simulink model "Project_Task1_4328802_SinghShrestha"  (Simulink 8.0)
settings: Solver=ode45  StartTime=0.0  StopTime=180*Ts  RelTol=1e-3
PreLoadFcn:
  | Ts=20e-9; % Sample period
  | W=9;        % Bit-width
  | 
  | n_constant = 109;
  | gap = 300;
  | 
  | % Input sequence for n signal
  | n_value = [0 n_constant zeros(1,gap)]';   %value
  | n_time = [0:length(n_value)-1]'*Ts;          % time
  | n = [n_time n_value];                                % signal
  | 
  | % Input sequence for start signal
  | start_value = [0 1 zeros(1,gap)]';                 % value
  | start_time = [0:length(start_value)-1]'*Ts;  % time
  | start = [start_time start_value];                  % signal
undefined symbols (not defined in the file): xlipgetpartsetting
libraries: xbsIndex_r4 x37
settings Model: Creator=alpha  LastModifiedBy=SaGuN MS
settings DataIOCC: SignalLoggingSaveFormat=ModelDataLogs
settings OptimizationCC: InitFltsAndDblsToZero=on
settings DebuggingCC: SaveWithParameterizedLinksMsg=none  SignalResolutionControl=TryResolveAllWithWarning  MultiTaskDSMMsg=warning  MultiTaskCondExecSysMsg=none  FcnCallInpInsideContextMsg=EnableAllAsWarning  StrictBusMsg=Warning
settings RTWCC: IncludeERTFirstTime=on
settings GRTTargetCC: TargetFcnLib=ansi_tfl_tmw.mat  CombineOutputUpdateFcns=off  GRTInterface=on

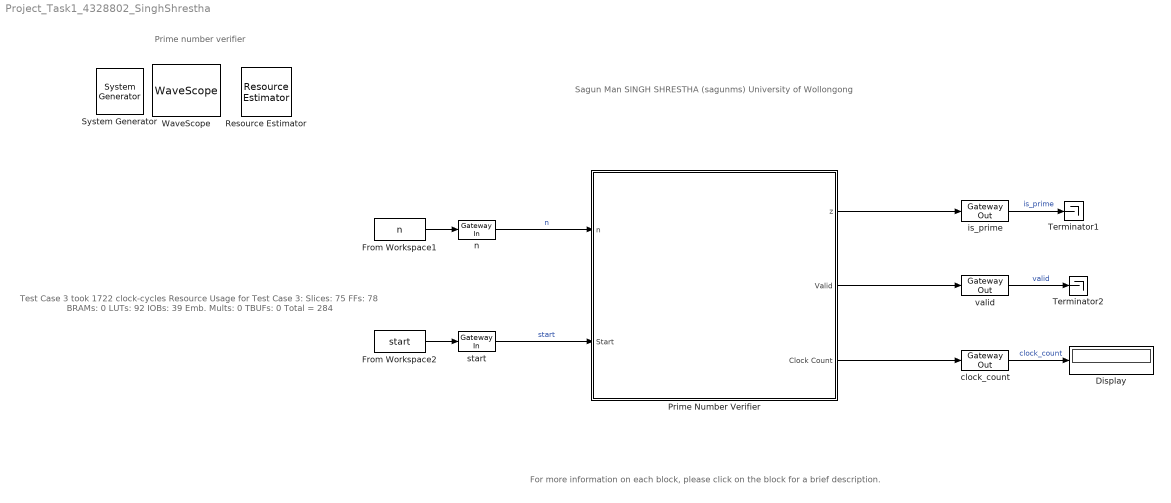
== system Project_Task1_4328802_SinghShrestha ==
  note: Prime number verifier
  note: Sagun Man SINGH SHRESTHA
      | (sagunms)
      | University of Wollongong
  note: Test Case 3 took 1722 clock-cycles
      |
      | Resource Usage for Test Case 3:
      | Slices: 75
      | FFs: 78
      | BRAMs: 0
      | LUTs: 92
      | IOBs: 39
      | Emb. Mults: 0
      | TBUFs: 0
      | Total = 284
  note: For more information on each block, please click on the block for a brief description.
  " System Generator" : xbsIndex_r4/ System Generator  Tag=genX  xilinxfamily=spartan3e  part=xc3s500e  speed=-4  package=fg320  synthesis_tool=XST  clock_wrapper=Clock Enables  directory=./ise  proj_type=Project Navigator  Synth_file=XST Defaults  Impl_file=ISE Defaults  testbench=off  simulink_period=Ts  sysclk_period=20  dcm_input_clock_period=100  incr_netlist=off  trim_vbits=Everywhere in SubSystem  dbl_ovrd=According to Block Masks  core_generation=According to Block Masks  run_coregen=off  deprecated_control=off  eval_field=0  block_type=sysgen
      settings: block_version=8.2.02
  Display : Display
  From Workspace1 : FromWorkspace  VariableName=n  SampleTime=Ts  Interpolate=off  OutputAfterFinalValue=Holding final value
  From Workspace2 : FromWorkspace  VariableName=start  SampleTime=Ts  Interpolate=off  OutputAfterFinalValue=Holding final value
  Prime Number Verifier : Subsystem
  Resource Estimator : xbsIndex_r4/Resource Estimator  Tag=resEstTag  Slices=75  FFs=78  BRAMs=0  LUTs=92  IOBs=39  EBMs=0  TBUFs=0  xl_use_estimator_area=off  est_options=Estimate  xl_estimator_area="[ 75  78   0  92  39   0   0 ]"  block_type=resource_estimator
      settings: AttributesFormatString=Resource\nEstimator  block_version=11.4
  Terminator1 : Terminator
  Terminator2 : Terminator
  WaveScope : xbsIndex_r4/WaveScope  block_type=wavescope
      settings: block_version=8.2.02
  clock_count : xbsIndex_r4/Gateway Out  inherit_from_input=off  hdl_port=on  timing_constraint=None  locs_specified=off  LOCs={'F9'}  UseAsDAC=off  DACChannel='1'  block_type=gatewayout
      settings: infoedit="Gateway out block.  Converts Xilinx fixed point inputs into ouputs of type Simulink integer, double, or fixed point.<P><P>Hardware notes:  In hardware these blocks become top level output ports or are discarded, depending on how they are configured."  xl_area=[0 0 0 0 24 0 0]  block_version=8.2.02
  is_prime : xbsIndex_r4/Gateway Out  inherit_from_input=off  hdl_port=on  timing_constraint=None  locs_specified=off  LOCs={'F9'}  UseAsDAC=off  DACChannel='1'  block_type=gatewayout
      settings: infoedit="Gateway out block.  Converts Xilinx fixed point inputs into ouputs of type Simulink integer, double, or fixed point.<P><P>Hardware notes:  In hardware these blocks become top level output ports or are discarded, depending on how they are configured."  xl_area=[0 0 0 0 1 0 0]  block_version=8.2.02
  n : xbsIndex_r4/Gateway In  gui_display_data_type=Fixed-point  arith_type=Unsigned  n_bits=W  bin_pt=0  preci_type=Single  exp_width=8  frac_width=24  quantization="Round  (unbiased: +/- Inf)"  overflow=Wrap  period=Ts  dbl_ovrd=off  timing_constraint=None  locs_specified=off  LOCs={'V16'}  UseAsADC=off  ADCChannel='1'  inherit_from_input=off  hdl_port=on  block_type=gatewayin
      settings: infoedit="Gateway in block.  Converts inputs of type Simulink integer, double and fixed point to  Xilinx fixed point type.<br><br>Hardware notes:  In hardware these blocks become top level input ports."  xl_area=[0 0 0 0 12 0 0]  block_version=8.2.02
  start : xbsIndex_r4/Gateway In  gui_display_data_type=Fixed-point  arith_type=Boolean  n_bits=W  bin_pt=0  preci_type=Single  exp_width=8  frac_width=24  quantization="Round  (unbiased: +/- Inf)"  overflow=Wrap  period=Ts  dbl_ovrd=off  timing_constraint=None  locs_specified=off  LOCs={'V16'}  UseAsADC=off  ADCChannel='1'  inherit_from_input=off  hdl_port=on  block_type=gatewayin
      settings: infoedit="Gateway in block.  Converts inputs of type Simulink integer, double and fixed point to  Xilinx fixed point type.<P><P>Hardware notes:  In hardware these blocks become top level input ports."  xl_area=[0 0 0 0 1 0 0]  block_version=8.2.02
  valid : xbsIndex_r4/Gateway Out  inherit_from_input=off  hdl_port=on  timing_constraint=None  locs_specified=off  LOCs={'F9'}  UseAsDAC=off  DACChannel='1'  block_type=gatewayout
      settings: infoedit="Gateway out block.  Converts Xilinx fixed point inputs into ouputs of type Simulink integer, double, or fixed point.<P><P>Hardware notes:  In hardware these blocks become top level output ports or are discarded, depending on how they are configured."  xl_area=[0 0 0 0 1 0 0]  block_version=8.2.02
  wires:
  From Workspace1/1 -> n/1
  From Workspace2/1 -> start/1
  is_prime/1 -> Terminator1/1  "is_prime"
  valid/1 -> Terminator2/1  "valid"
  clock_count/1 -> Display/1  "clock_count"
  n/1 -> Prime Number Verifier/1(n)  "n"
  start/1 -> Prime Number Verifier/2(Start)  "start"
  Prime Number Verifier/1(z) -> is_prime/1
  Prime Number Verifier/2(Valid) -> valid/1
  Prime Number Verifier/3(Clock Count) -> clock_count/1

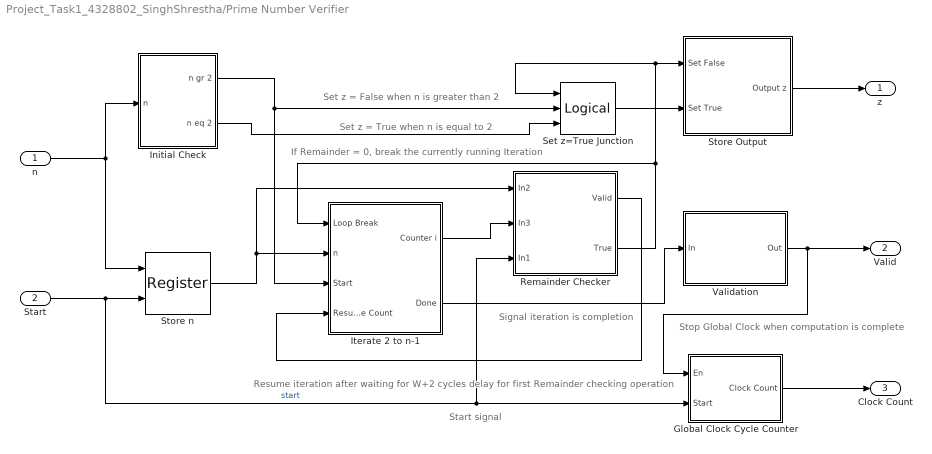
== system Project_Task1_4328802_SinghShrestha/Prime Number Verifier ==
  note: Start signal
  note: Set z = False when n is greater than 2
  note: Set z = True when n is equal to 2
  note: Signal iteration is completion
  note: If Remainder = 0, break the currently running Iteration
  note: Resume iteration after waiting for W+2 cycles delay for first Remainder checking operation
  note: Stop Global Clock when computation is complete
  n : Inport
  Start : Inport  Port=2
  Global Clock Cycle Counter : Subsystem
  Initial Check : Subsystem
  Iterate 2 to n-1 : Subsystem
  Remainder Checker : Subsystem
  Set z=True Junction : xbsIndex_r4/Logical  logical_function=OR  inputs=3  en=off  latency=0  precision=Full  arith_type=Unsigned  n_bits=16  bin_pt=0  align_bp=on  dbl_ovrd=off  block_type=logical
      settings: xl_area=[1 0 0 1 0 0 0]
  Store Output : Subsystem
  Store n : xbsIndex_r4/Register  init=0  rst=off  en=on  dbl_ovrd=off  block_type=register
      settings: xl_area=[6 12 0 0 0 0 0]
  Validation : Subsystem
  z : Outport
  Valid : Outport  Port=2
  Clock Count : Outport  Port=3
  wires:
  Start/1 -> Global Clock Cycle Counter/2(Start), Remainder Checker/3(In1), Store n/2  "start"
  n/1 -> Store n/1, Initial Check/1(n)
  Store n/1 -> Remainder Checker/1(In2), Iterate 2 to n-1/2(n)
  Validation/1(Out) -> Global Clock Cycle Counter/1(En), Valid/1
  Global Clock Cycle Counter/1(Clock Count) -> Clock Count/1
  Initial Check/1(n gr 2) -> Set z=True Junction/2, Iterate 2 to n-1/3(Start)
  Store Output/1(Output z) -> z/1
  Initial Check/2(n eq 2) -> Set z=True Junction/3
  Set z=True Junction/1 -> Store Output/2(Set True)
  Iterate 2 to n-1/2(Done) -> Validation/1(In)
  Remainder Checker/2(True) -> Store Output/1(Set False), Set z=True Junction/1, Iterate 2 to n-1/1(Loop Break)
  Iterate 2 to n-1/1(Counter i) -> Remainder Checker/2(In3)
  Remainder Checker/1(Valid) -> Iterate 2 to n-1/4(Resume Count)

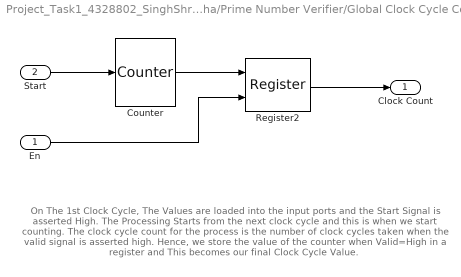
== system Project_Task1_4328802_SinghShrestha/Prime Number Verifier/Global Clock Cycle Counter ==
  note: On The 1st Clock Cycle, The Values are loaded into the input ports and the Start Signal is asserted High.
      |
      | The Processing Starts from the next clock cycle and this is when we start counting.
      | The clock cycle count for the process is the number of clock cycles taken when the valid signal is asserted high.
      |
      | Hence, we store the value of the counter when Valid=High in a register and This becomes our final Clock Cycle Value.
  En : Inport
  Start : Inport  Port=2
  Counter : xbsIndex_r4/Counter  cnt_type=Free Running  cnt_to=Inf  operation=Up  start_count=1  cnt_by_val=1  arith_type=Unsigned  n_bits=2*W  bin_pt=0  load_pin=off  rst=on  en=off  explicit_period=off  period=1  dbl_ovrd=off  use_behavioral_HDL=off  implementation=Fabric  use_rpm=off  block_type=counter
      settings: xl_area=[13 24 0 24 0 0 0]  block_version=8.2.02
  Register2 : xbsIndex_r4/Register  init=0  rst=off  en=on  dbl_ovrd=off  block_type=register
      settings: xl_area=[12 24 0 0 0 0 0]  block_version=11.4
  Clock Count : Outport
  wires:
  Counter/1 -> Register2/1
  Register2/1 -> Clock Count/1
  Start/1 -> Counter/1
  En/1 -> Register2/2

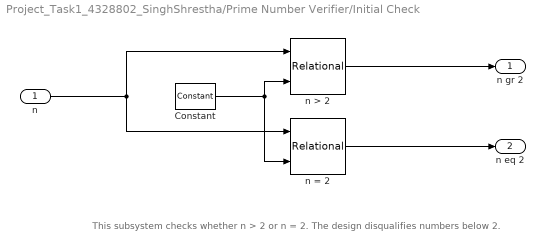
== system Project_Task1_4328802_SinghShrestha/Prime Number Verifier/Initial Check ==
  note: This subsystem checks whether n > 2 or n = 2. The design disqualifies numbers below 2.
  n : Inport
  Constant : xbsIndex_r4/Constant  const=2  gui_display_data_type=Fixed-point  arith_type=Unsigned  n_bits=2  bin_pt=0  preci_type=Single  exp_width=8  frac_width=24  explicit_period=off  period=1  equ=P=C  opselect=C  inp2=PCIN>>17  opr=+  inp1=P  carry=CIN  dbl_ovrd=off  block_type=constant
  n = 2 : xbsIndex_r4/Relational  mode=a=b  en=off  latency=0  dbl_ovrd=off  block_type=relational
      settings: xl_area=[3 0 0 6 0 0 0]
  n > 2 : xbsIndex_r4/Relational  mode=a>b  en=off  latency=0  dbl_ovrd=off  block_type=relational
      settings: xl_area=[6 0 0 12 0 0 0]
  n gr 2 : Outport
  n eq 2 : Outport  Port=2
  wires:
  n > 2/1 -> n gr 2/1
  Constant/1 -> n > 2/2, n = 2/2
  n = 2/1 -> n eq 2/1
  n/1 -> n > 2/1, n = 2/1

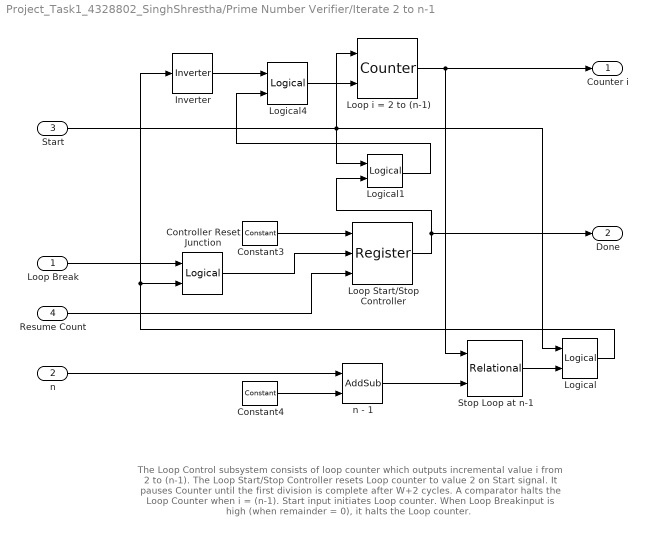
== system Project_Task1_4328802_SinghShrestha/Prime Number Verifier/Iterate 2 to n-1 ==
  note: The Loop Control subsystem consists of loop counter which outputs incremental value i from 2 to (n-1).
      | The Loop Start/Stop Controller resets Loop counter to value 2 on Start signal. It pauses Counter until the first division is complete after W+2 cycles.
      | A comparator halts the Loop Counter when i = (n-1).
      |
      | Start input initiates Loop counter. When Loop Breakinput is high (when remainder = 0), it halts the Loop counter.
  Loop Break : Inport
  n : Inport  Port=2
  Start : Inport  Port=3
  Resume Count : Inport  Port=4
  Constant3 : xbsIndex_r4/Constant  const=1  gui_display_data_type=Boolean  arith_type=Boolean  n_bits=16  bin_pt=14  preci_type=Single  exp_width=8  frac_width=24  explicit_period=off  period=1  equ=P=C  opselect=C  inp2=PCIN>>17  opr=+  inp1=P  carry=CIN  dbl_ovrd=off  block_type=constant
  Constant4 : xbsIndex_r4/Constant  const=1  gui_display_data_type=Fixed-point  arith_type=Unsigned  n_bits=W  bin_pt=0  preci_type=Single  exp_width=8  frac_width=24  explicit_period=off  period=1  equ=P=C  opselect=C  inp2=PCIN>>17  opr=+  inp1=P  carry=CIN  dbl_ovrd=off  block_type=constant
  Controller Reset Junction : xbsIndex_r4/Logical  logical_function=OR  inputs=2  en=off  latency=0  precision=Full  arith_type=Unsigned  n_bits=16  bin_pt=0  align_bp=on  dbl_ovrd=off  block_type=logical
      settings: xl_area=[1 0 0 1 0 0 0]
  Inverter : xbsIndex_r4/Inverter  en=off  latency=0  dbl_ovrd=off  block_type=inv
      settings: xl_area=[0 0 0 0 0 0 0]
  Logical : xbsIndex_r4/Logical  logical_function=NOR  inputs=2  en=off  latency=0  precision=Full  arith_type=Unsigned  n_bits=16  bin_pt=0  align_bp=on  dbl_ovrd=off  block_type=logical
      settings: xl_area=[1 0 0 1 0 0 0]
  Logical1 : xbsIndex_r4/Logical  logical_function=OR  inputs=2  en=off  latency=0  precision=Full  arith_type=Unsigned  n_bits=16  bin_pt=0  align_bp=on  dbl_ovrd=off  block_type=logical
      settings: xl_area=[1 0 0 1 0 0 0]
  Logical4 : xbsIndex_r4/Logical  logical_function=AND  inputs=2  en=off  latency=0  precision=Full  arith_type=Unsigned  n_bits=16  bin_pt=0  align_bp=on  dbl_ovrd=off  block_type=logical
      settings: xl_area=[1 0 0 1 0 0 0]
  Loop Start/Stop Controller : xbsIndex_r4/Register  init=0  rst=on  en=on  dbl_ovrd=off  block_type=register
      settings: xl_area=[1 1 0 0 0 0 0]
  Loop i = 2 to (n-1) : xbsIndex_r4/Counter  cnt_type=Free Running  cnt_to=Inf  operation=Up  start_count=2  cnt_by_val=1  arith_type=Unsigned  n_bits=W  bin_pt=0  load_pin=off  rst=on  en=on  explicit_period=off  period=1  dbl_ovrd=off  use_behavioral_HDL=off  implementation=Fabric  block_type=counter
      settings: xl_area=[7 12 0 12 0 0 0]
  Stop Loop at n-1 : xbsIndex_r4/Relational  mode=a<b  en=off  latency=0  dbl_ovrd=off  block_type=relational
      settings: xl_area=[7 0 0 13 0 0 0]
  n - 1 : xbsIndex_r4/AddSub  mode=Subtraction  use_carryin=off  use_carryout=off  en=off  latency=0  precision=Full  arith_type=Unsigned  n_bits=16  bin_pt=14  quantization=Truncate  overflow=Wrap  dbl_ovrd=off  use_behavioral_HDL=off  hw_selection=Fabric  pipelined=off  block_type=addsub
      settings: xl_area=[7 0 0 12 0 0 0]
  Counter i : Outport
  Done : Outport  Port=2
  wires:
  n - 1/1 -> Stop Loop at n-1/2
  Inverter/1 -> Logical4/1
  Constant3/1 -> Loop Start/Stop Controller/1
  Logical/1 -> Inverter/1, Controller Reset Junction/2
  Loop i = 2 to (n-1)/1 -> Counter i/1, Stop Loop at n-1/1
  Controller Reset Junction/1 -> Loop Start/Stop Controller/2
  Constant4/1 -> n - 1/2
  Logical4/1 -> Loop i = 2 to (n-1)/2
  Logical1/1 -> Logical4/2
  Loop Break/1 -> Controller Reset Junction/1
  Start/1 -> Logical/1, Loop i = 2 to (n-1)/1, Logical1/1
  Resume Count/1 -> Loop Start/Stop Controller/3
  Loop Start/Stop Controller/1 -> Done/1, Logical1/2
  n/1 -> n - 1/1
  Stop Loop at n-1/1 -> Logical/2

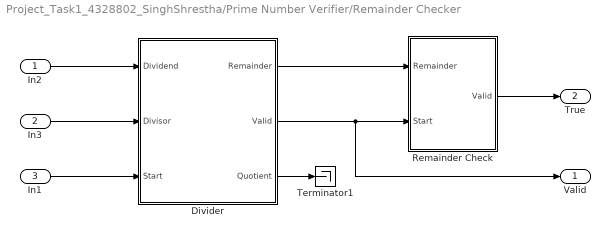
== system Project_Task1_4328802_SinghShrestha/Prime Number Verifier/Remainder Checker ==
  In2 : Inport
  In3 : Inport  Port=2
  In1 : Inport  Port=3
  Divider : Subsystem
  Remainder Check : Subsystem
  Terminator1 : Terminator
  Valid : Outport
  True : Outport  Port=2
  wires:
  Divider/3(Quotient) -> Terminator1/1
  In1/1 -> Divider/3(Start)
  In2/1 -> Divider/1(Dividend)
  Divider/2(Valid) -> Remainder Check/2(Start), Valid/1
  Divider/1(Remainder) -> Remainder Check/1(Remainder)
  Remainder Check/1(Valid) -> True/1
  In3/1 -> Divider/2(Divisor)

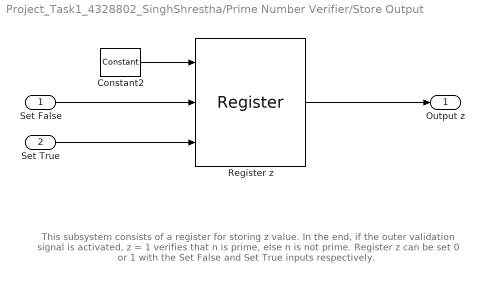
== system Project_Task1_4328802_SinghShrestha/Prime Number Verifier/Store Output ==
  note: This subsystem consists of a register for storing z value.
      | In the end, if the outer validation signal is activated, z = 1 verifies that n is prime, else n is not prime.
      | Register z can be set 0 or 1 with the Set False and Set True inputs respectively.
  Set False : Inport
  Set True : Inport  Port=2
  Constant2 : xbsIndex_r4/Constant  const=1  gui_display_data_type=Boolean  arith_type=Boolean  n_bits=16  bin_pt=14  preci_type=Single  exp_width=8  frac_width=24  explicit_period=off  period=1  equ=P=C  opselect=C  inp2=PCIN>>17  opr=+  inp1=P  carry=CIN  dbl_ovrd=off  block_type=constant
  Register z : xbsIndex_r4/Register  init=0  rst=on  en=on  dbl_ovrd=off  block_type=register
      settings: xl_area=[1 1 0 0 0 0 0]
  Output z : Outport
  wires:
  Constant2/1 -> Register z/1
  Register z/1 -> Output z/1
  Set True/1 -> Register z/3
  Set False/1 -> Register z/2

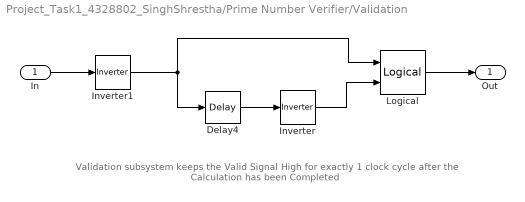
== system Project_Task1_4328802_SinghShrestha/Prime Number Verifier/Validation ==
  note: Validation subsystem keeps the Valid Signal High for exactly 1 clock cycle
      | after the Calculation has been Completed
  In : Inport
  Delay4 : xbsIndex_r4/Delay  rst=off  infoeditControl=Selection of Reset will increase slice count due to use of real FFs and instead of SRLs  en=off  latency=1  dbl_ovrd=off  reg_retiming=off  block_type=delay
      settings: infoedit=Hardware notes: A delay line is a chain, each link of which is an SRL16 followed by a flip-flop. If register retiming is enabled, the delay line is a chain of flip-flops.  xl_area=[1 1 0 0 0 0 0]  block_version=8.2.02
  Inverter : xbsIndex_r4/Inverter  en=off  latency=0  dbl_ovrd=off  block_type=inv
      settings: xl_area=[0 0 0 0 0 0 0]  block_version=11.4
  Inverter1 : xbsIndex_r4/Inverter  en=off  latency=0  dbl_ovrd=off  block_type=inv
      settings: xl_area=[0 0 0 0 0 0 0]
  Logical : xbsIndex_r4/Logical  logical_function=AND  inputs=2  en=off  latency=0  precision=Full  arith_type=Unsigned  n_bits=16  bin_pt=0  align_bp=on  dbl_ovrd=off  block_type=logical
      settings: xl_area=[1 0 0 1 0 0 0]  block_version=11.4
  Out : Outport
  wires:
  Inverter/1 -> Logical/2
  Delay4/1 -> Inverter/1
  Logical/1 -> Out/1
  Inverter1/1 -> Logical/1, Delay4/1
  In/1 -> Inverter1/1

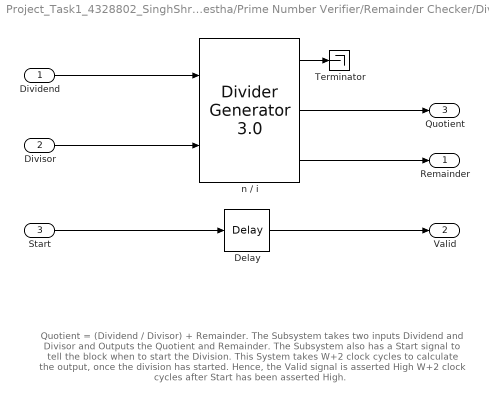
== system Project_Task1_4328802_SinghShrestha/Prime Number Verifier/Remainder Checker/Divider ==
  note: Quotient = (Dividend / Divisor) + Remainder.
      |
      | The Subsystem takes two inputs Dividend and Divisor and Outputs the Quotient and Remainder.
      | The Subsystem also has a Start signal to tell the block when to start the Division.
      |
      | This System takes W+2 clock cycles to calculate the output, once the division has started.
      | Hence, the Valid signal is asserted High W+2 clock cycles after Start has been asserted High.
  Dividend : Inport
  Divisor : Inport  Port=2
  Start : Inport  Port=3
  Delay : xbsIndex_r4/Delay  rst=off  infoeditControl=Selection of Reset will increase slice count due to use of real FFs and instead of SRLs  en=off  latency=W+2  dbl_ovrd=off  reg_retiming=off  block_type=delay
      settings: xl_area=[1 1 0 1 0 0 0]
  Terminator : Terminator
  n / i : xbsIndex_r4/Divider Generator 3.0   dividend_and_quotient_width=W  divisor_width=W  algorithm_type=Radix2  remainder_type=Remainder  fractional_width=32  clocks_per_division=1  divide_by_zero_detect=off  latency_configuration=Automatic  latency=6  ce=off  sclr=off  sclr_ce_priority=SCLR_overrides_CE  operand_sign=Signed  ip_name=Divider Generator  ip_version=3.0  dsptool_ready=true  wrapper_available=true  port_translation_map={ 'ce' => 'en', 'sclr' => 'rst' }  ipcore_fpga_part=xlipgetpartsetting(gcb, {'virtex4', 'xc4vsx35', '-10', 'ff668'})  ipcore_verbose=false  block_type=div_gen_v3_0
  Remainder : Outport
  Valid : Outport  Port=2
  Quotient : Outport  Port=3
  wires:
  n / i/1 -> Terminator/1
  n / i/3 -> Remainder/1
  Delay/1 -> Valid/1
  Divisor/1 -> n / i/2
  Start/1 -> Delay/1
  Dividend/1 -> n / i/1
  n / i/2 -> Quotient/1

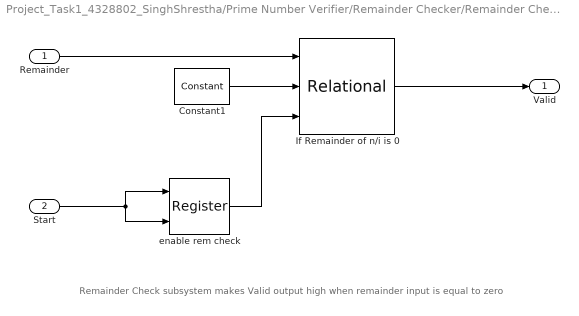
== system Project_Task1_4328802_SinghShrestha/Prime Number Verifier/Remainder Checker/Remainder Check ==
  note: Remainder Check subsystem makes Valid output high when remainder input is equal to zero
  Remainder : Inport
  Start : Inport  Port=2
  Constant1 : xbsIndex_r4/Constant  const=0  gui_display_data_type=Fixed-point  arith_type=Unsigned  n_bits=W  bin_pt=0  preci_type=Single  exp_width=8  frac_width=24  explicit_period=off  period=1  equ=P=C  opselect=C  inp2=PCIN>>17  opr=+  inp1=P  carry=CIN  dbl_ovrd=off  block_type=constant
  If Remainder of n/i is 0 : xbsIndex_r4/Relational  mode=a=b  en=on  latency=1  dbl_ovrd=off  block_type=relational
      settings: xl_area=[3 1 0 6 0 0 0]
  enable rem check : xbsIndex_r4/Register  init=0  rst=off  en=on  dbl_ovrd=off  block_type=register
      settings: xl_area=[1 1 0 0 0 0 0]
  Valid : Outport
  wires:
  Constant1/1 -> If Remainder of n/i is 0/2
  enable rem check/1 -> If Remainder of n/i is 0/3
  If Remainder of n/i is 0/1 -> Valid/1
  Remainder/1 -> If Remainder of n/i is 0/1
  Start/1 -> enable rem check/1, enable rem check/2
